simulink model "DecentralizedPID"  (R2024b)
settings: Solver=VariableStepAuto  StartTime=0.0  StopTime=20  RelTol=1e-3
libraries: Mako_Dynamics x1
settings Model: Creator=pinto  LastModifiedBy=pinto

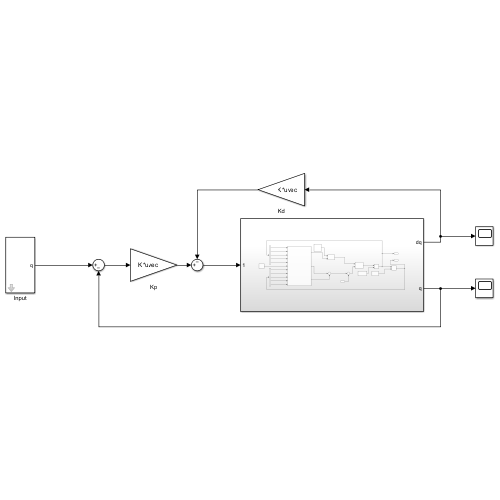
[thumbnail: Simulink's stored preview of the top-level diagram]
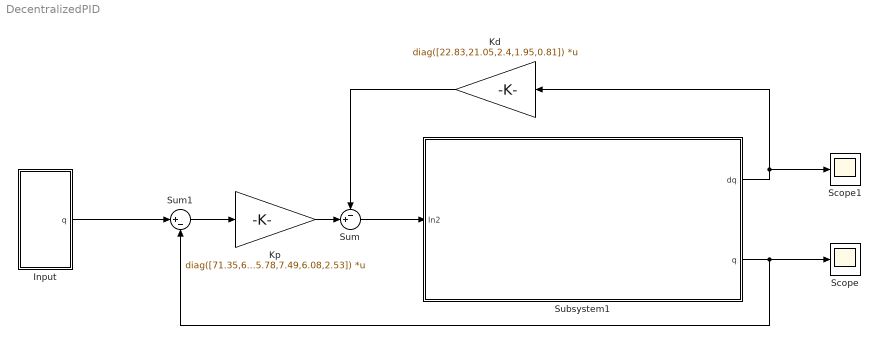
== system DecentralizedPID ==
  Input : Subsystem  mask{q1=50.400, q2=39.600, q3=25.200, q4=68.400, q5=108.0, q6=-54.0}
  Kd : Gain  Gain=diag([22.83,21.05,2.4,1.95,0.81])  Multiplication=Matrix(K*u) (u vector)
  Kp : Gain  Gain=diag([71.35,65.78,7.49,6.08,2.53])  Multiplication=Matrix(K*u) (u vector)
  Scope : Scope
  Scope1 : Scope
  Subsystem1 : Subsystem
  Sum : Sum  Inputs=-+|
  Sum1 : Sum  Inputs=|+-
  wires:
  Kd/1 -> Sum/1
  Subsystem1/2(q) -> Scope/1, Sum1/2
  Sum/1 -> Subsystem1/1(In2)
  Kp/1 -> Sum/2
  Sum1/1 -> Kp/1
  Subsystem1/1(dq) -> Scope1/1, Kd/1
  Input/1(q) -> Sum1/1

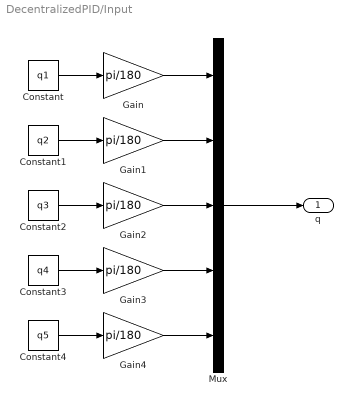
== system DecentralizedPID/Input ==
  Constant : Constant  Value=q1
  Constant1 : Constant  Value=q2
  Constant2 : Constant  Value=q3
  Constant3 : Constant  Value=q4
  Constant4 : Constant  Value=q5
  Gain{,1..4} (5 alike) : Gain  Gain=pi/180
  Mux : Mux  Inputs=5
  q : Outport
  wires:
  Constant/1 -> Gain/1
  Gain/1 -> Mux/1
  Mux/1 -> q/1
  Gain1/1 -> Mux/2
  Constant1/1 -> Gain1/1
  Gain2/1 -> Mux/3
  Constant2/1 -> Gain2/1
  Constant3/1 -> Gain3/1
  Gain3/1 -> Mux/4
  Constant4/1 -> Gain4/1
  Gain4/1 -> Mux/5

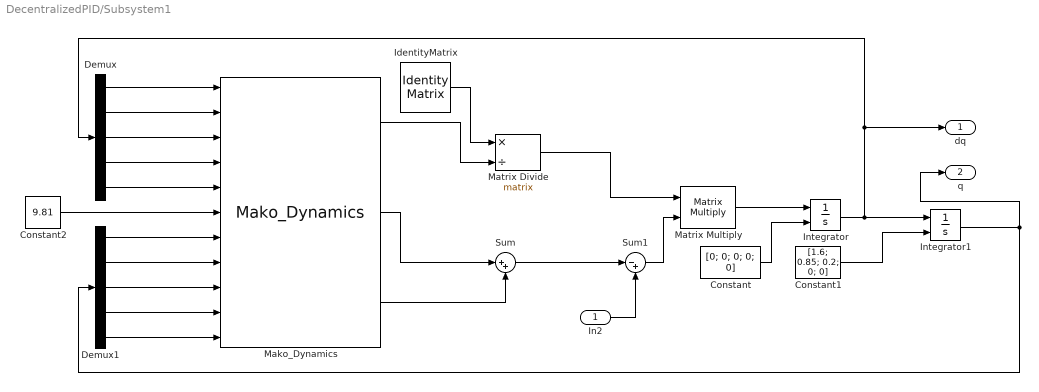
== system DecentralizedPID/Subsystem1 ==
  In2 : Inport
  Constant : Constant  Value=[0; 0; 0; 0; 0]
  Constant1 : Constant  Value=[1.6; 0.85; 0.2; 0; 0]
  Constant2 : Constant  Value=9.81
  Demux : Demux  Outputs=5
  Demux1 : Demux  Outputs=5
  IdentityMatrix : IdentityMatrix
  Integrator : Integrator  InitialConditionSource=external  InitialCondition=[0.01, 0.01, 0.01]
  Integrator1 : Integrator  InitialConditionSource=external  InitialCondition=[0.01, 0.01, 0.01]
  Mako_Dynamics : Mako_Dynamics/Mako_Dynamics  SystemSampleTime=-1  VariantActivationTime=update diagram  AllowFlexibleInterface=on  Latency=0  AutoFrameSizeCalculation=off
  Matrix Divide : Product  Inputs=*/  Multiplication=Matrix(*)
  Matrix Multiply : Product  Multiplication=Matrix(*)
  Sum : Sum  Inputs=|++
  Sum1 : Sum  Inputs=|-+
  dq : Outport
  q : Outport  Port=2
  wires:
  Demux1/4 -> Mako_Dynamics/10
  Sum/1 -> Sum1/1
  Mako_Dynamics/3 -> Sum/2
  Demux/3 -> Mako_Dynamics/3
  IdentityMatrix/1 -> Matrix Divide/1
  Integrator/1 -> Integrator1/1, dq/1, Demux/1
  Matrix Multiply/1 -> Integrator/1
  Demux/4 -> Mako_Dynamics/4
  Demux1/1 -> Mako_Dynamics/7
  Demux1/5 -> Mako_Dynamics/11
  Demux/2 -> Mako_Dynamics/2
  Constant1/1 -> Integrator1/2
  Integrator1/1 -> q/1, Demux1/1
  Mako_Dynamics/1 -> Matrix Divide/2
  Matrix Divide/1 -> Matrix Multiply/1
  Constant/1 -> Integrator/2
  Demux1/2 -> Mako_Dynamics/8
  Constant2/1 -> Mako_Dynamics/6
  Sum1/1 -> Matrix Multiply/2
  Demux/1 -> Mako_Dynamics/1
  In2/1 -> Sum1/2
  Mako_Dynamics/2 -> Sum/1
  Demux/5 -> Mako_Dynamics/5
  Demux1/3 -> Mako_Dynamics/9
